simulink model "Ex_Sep_2020_A"  (R2022b)
settings: Solver=VariableStepAuto  StartTime=0.0  StopTime=150  RelTol=1e-3
settings Model: Creator=rrilo  LastModifiedBy=rrilo

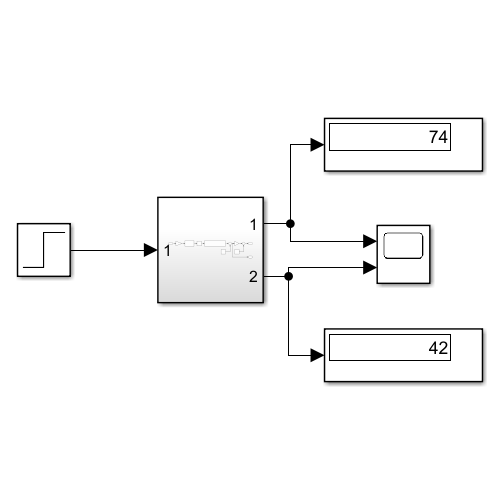
[thumbnail: Simulink's stored preview of the top-level diagram]
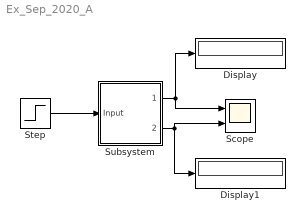
== system Ex_Sep_2020_A ==
  Display : Display
  Display1 : Display
  Scope : Scope  NumInputPorts=2
  Step : Step  After=50  SampleTime=0
  Subsystem : Subsystem
  wires:
  Step/1 -> Subsystem/1(Input)
  Subsystem/1(Output) -> Scope/1, Display/1
  Subsystem/2(Output1) -> Display1/1, Scope/2

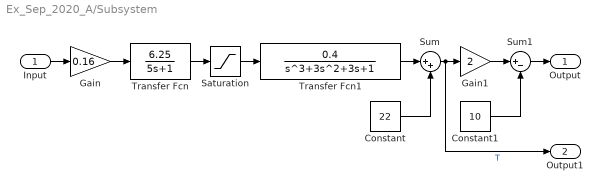
== system Ex_Sep_2020_A/Subsystem ==
  Input : Inport
  Constant : Constant  Value=22
  Constant1 : Constant  Value=10
  Gain : Gain  Gain=0.16
  Gain1 : Gain  Gain=2
  Saturation : Saturate  UpperLimit=100  LowerLimit=0
  Sum : Sum  Inputs=|++
  Sum1 : Sum  Inputs=|+-
  Transfer Fcn : TransferFcn  Numerator=[6.25]  Denominator=[5 1]
  Transfer Fcn1 : TransferFcn  Numerator=[0.4]  Denominator=[1 3 3 1]
  Output : Outport
  Output1 : Outport  Port=2
  wires:
  Constant1/1 -> Sum1/2
  Transfer Fcn1/1 -> Sum/1
  Saturation/1 -> Transfer Fcn1/1
  Input/1 -> Gain/1
  Constant/1 -> Sum/2
  Sum/1 -> Output1/1, Gain1/1  "T"
  Gain/1 -> Transfer Fcn/1
  Gain1/1 -> Sum1/1
  Transfer Fcn/1 -> Saturation/1
  Sum1/1 -> Output/1
